simulink model "robot_3axis"  (R2024b)
settings: Solver=ode4  StartTime=0.0  StopTime=simulation_time  FixedStep=Ts  RelTol=1e-3
undefined symbols (not defined in the file): b_r, b_theta, b_z, d_r, d_theta, d_z, dff_r, dff_theta, dff_z, disturbance_time, F_r_max, F_z_max, F_z_min, ff_enable, g, gravity_comp, J_theta, Kd_r, Kd_theta, Kd_z, Ki_r, Ki_theta, Ki_z, Kp_r, Kp_theta, Kp_z, m_r, m_z, move_time, N_filter, noise_r, noise_theta, noise_z, plant_mass_scale, r_final, r_initial, T_theta_max, theta_final, theta_initial, Ts, z_final, z_initial
libraries: slpidlib x3
settings Model: Creator=dell  LastModifiedBy=dell

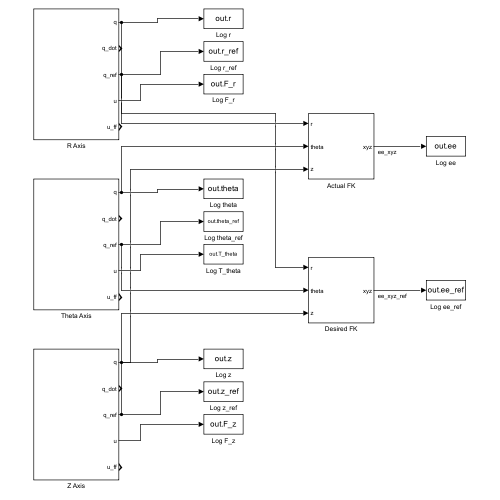
[thumbnail: Simulink's stored preview of the top-level diagram]
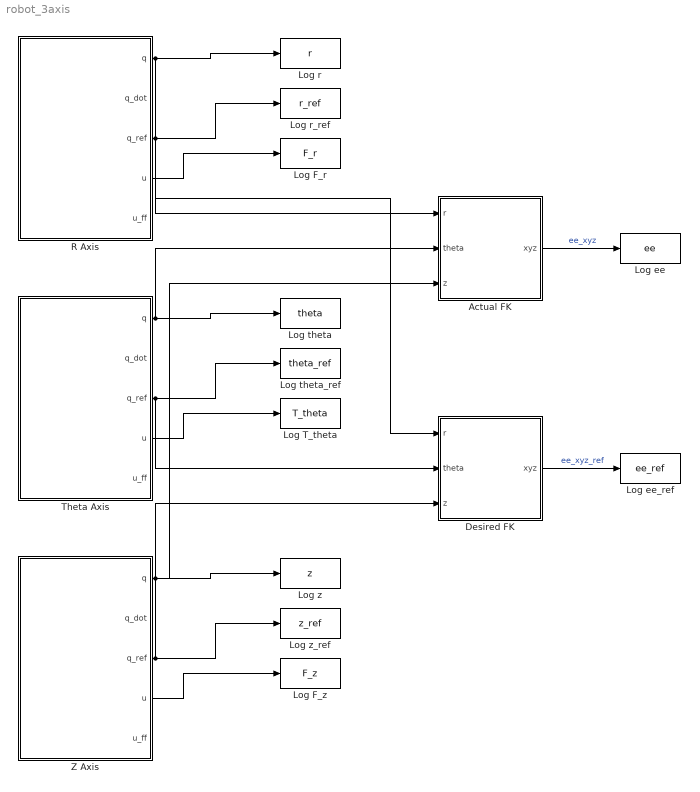
== system robot_3axis ==
  Actual FK : Subsystem
  Desired FK : Subsystem
  Log F_r : ToWorkspace  VariableName=F_r  SaveFormat=Timeseries  SampleTime=-1
  Log F_z : ToWorkspace  VariableName=F_z  SaveFormat=Timeseries  SampleTime=-1
  Log T_theta : ToWorkspace  VariableName=T_theta  SaveFormat=Timeseries  SampleTime=-1
  Log ee : ToWorkspace  VariableName=ee  SaveFormat=Timeseries  SampleTime=-1
  Log ee_ref : ToWorkspace  VariableName=ee_ref  SaveFormat=Timeseries  SampleTime=-1
  Log r : ToWorkspace  VariableName=r  SaveFormat=Timeseries  SampleTime=-1
  Log r_ref : ToWorkspace  VariableName=r_ref  SaveFormat=Timeseries  SampleTime=-1
  Log theta : ToWorkspace  VariableName=theta  SaveFormat=Timeseries  SampleTime=-1
  Log theta_ref : ToWorkspace  VariableName=theta_ref  SaveFormat=Timeseries  SampleTime=-1
  Log z : ToWorkspace  VariableName=z  SaveFormat=Timeseries  SampleTime=-1
  Log z_ref : ToWorkspace  VariableName=z_ref  SaveFormat=Timeseries  SampleTime=-1
  R Axis : Subsystem
  Theta Axis : Subsystem
  Z Axis : Subsystem
  wires:
  R Axis/1(q) -> Log r/1, Actual FK/1(r)
  R Axis/3(q_ref) -> Log r_ref/1, Desired FK/1(r)
  R Axis/4(u) -> Log F_r/1
  Theta Axis/1(q) -> Log theta/1, Actual FK/2(theta)
  Theta Axis/3(q_ref) -> Log theta_ref/1, Desired FK/2(theta)
  Theta Axis/4(u) -> Log T_theta/1
  Z Axis/1(q) -> Log z/1, Actual FK/3(z)
  Z Axis/3(q_ref) -> Log z_ref/1, Desired FK/3(z)
  Z Axis/4(u) -> Log F_z/1
  Actual FK/1(xyz) -> Log ee/1  "ee_xyz"
  Desired FK/1(xyz) -> Log ee_ref/1  "ee_xyz_ref"

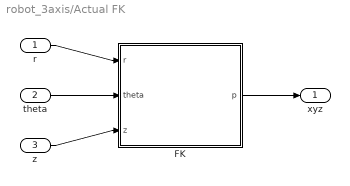
== system robot_3axis/Actual FK ==
  r : Inport
  theta : Inport  Port=2
  z : Inport  Port=3
  FK : MATLAB Function  TreatAsAtomicUnit=on
  xyz : Outport
  wires:
  r/1 -> FK/1(r)
  theta/1 -> FK/2(theta)
  z/1 -> FK/3(z)
  FK/1(p) -> xyz/1

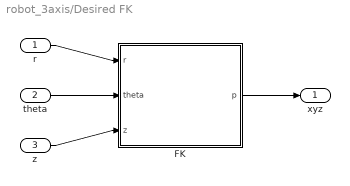
== system robot_3axis/Desired FK ==
  r : Inport
  theta : Inport  Port=2
  z : Inport  Port=3
  FK : MATLAB Function  TreatAsAtomicUnit=on
  xyz : Outport
  wires:
  r/1 -> FK/1(r)
  theta/1 -> FK/2(theta)
  z/1 -> FK/3(z)
  FK/1(p) -> xyz/1

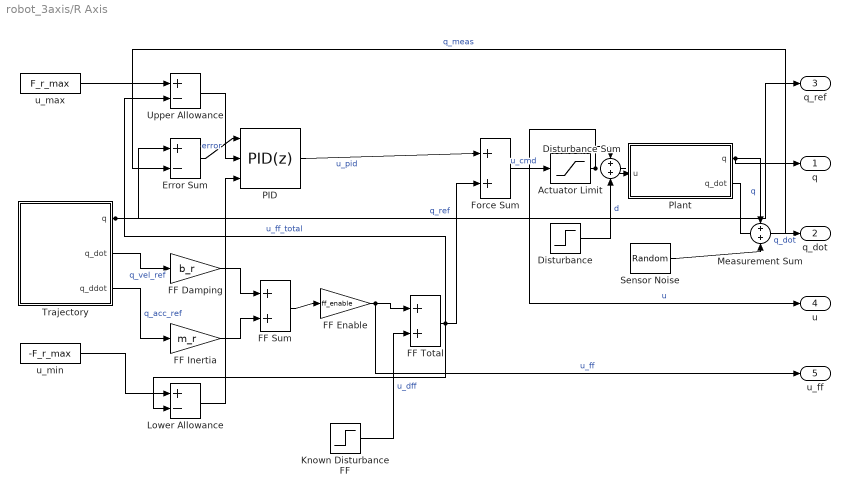
== system robot_3axis/R Axis ==
  Actuator Limit : Saturate  UpperLimit=F_r_max  LowerLimit=-F_r_max
  Disturbance : Step  Time=disturbance_time  After=d_r  SampleTime=0
  Disturbance Sum : Sum
  Error Sum : Sum  Inputs=+-
  FF Damping : Gain  Gain=b_r
  FF Enable : Gain  Gain=ff_enable
  FF Inertia : Gain  Gain=m_r
  FF Sum : Sum
  FF Total : Sum
  Force Sum : Sum
  Known Disturbance FF : Step  Time=disturbance_time  After=dff_r  SampleTime=0
  Lower Allowance : Sum  Inputs=+-
  Measurement Sum : Sum
  PID : slpidlib/PID Controller  Controller=PID  Form=Parallel  TimeDomain=Discrete-time  UseExternalTs=off  SampleTime=Ts  IntegratorMethod=Backward Euler  FilterMethod=Backward Euler  ControllerParametersSource=internal  P=Kp_r  I=Ki_r  UseKiTs=off  D=Kd_r  UseExternalDerivativeSource=off  N=N_filter  UseFilter=off  TunerSelectOption=Transfer Function Based (PID Tuner App)  InitialConditionSource=internal  InitialConditionForIntegrator=0  InitialConditionForFilter=0  DifferentiatorICPrevScaledInput=0  ExternalReset=none  TrackingMode=off  Kt=1  LimitOutput=on  SatLimitsSource=external  UpperSaturationLimit=inf  LowerSaturationLimit=-inf  LinearizeAsGain=off  AntiWindupMode=clamping  Kb=1  LimitIntegrator=off  UpperIntegratorSaturationLimit=inf  LowerIntegratorSaturationLimit=-inf  POutMin=[]  POutMax=[]  IOutMin=[]  IOutMax=[]  DOutMin=[]  DOutMax=[]  NOutMin=[]  NOutMax=[]  SumOutMin=[]  SumOutMax=[]  SaturationOutMin=[]  SaturationOutMax=[]  PParamMin=[]  PParamMax=[]  IParamMin=[]  IParamMax=[]  DParamMin=[]  DParamMax=[]  NParamMin=[]  NParamMax=[]  KbParamMin=[]  KbParamMax=[]  KtParamMin=[]  KtParamMax=[]  KbOutMin=[]  KbOutMax=[]  KtOutMin=[]  KtOutMax=[]  IntegratorOutMin=[]  IntegratorOutMax=[]  FilterOutMin=[]  FilterOutMax=[]  SumI1OutMin=[]  SumI1OutMax=[]  SumI2OutMin=[]  SumI2OutMax=[]  SumI3OutMin=[]  SumI3OutMax=[]  SumI4OutMin=[]  SumI4OutMax=[]  SumDOutMin=[]  SumDOutMax=[]  DifferentiatorOutMin=[]  DifferentiatorOutMax=[]  FilterDiffOutCoefMin=[]  FilterDiffOutCoefMax=[]  ReciprocalOutMin=[]  ReciprocalOutMax=[]  SumDenOutMin=[]  SumDenOutMax=[]  SumNumOutMin=[]  SumNumOutMax=[]  DivideOutMin=[]  DivideOutMax=[]  UdiffTsProdOutMin=[]  UdiffTsProdOutMax=[]  NTsProdOutMin=[]  NTsProdOutMax=[]  UintegralTsProdOutMin=[]  UintegralTsProdOutMax=[]  UngainTsProdOutMin=[]  UngainTsProdOutMax=[]  ClampingZeroOutDataTypeStr=Inherit: Inherit via back propagation  ClampingZeroOutMin=[]  ClampingZeroOutMax=[]  FilterDenConstantOutDataTypeStr=Inherit: Inherit via back propagation  FilterDenConstantOutMin=[]  FilterDenConstantOutMax=[]  PCopyOutDataTypeStr=Inherit: Inherit via back propagation  PCopyOutMin=[]  PCopyOutMax=[]  NCopyOutDataTypeStr=Inherit: Inherit via back propagation  NCopyOutMin=[]  NCopyOutMax=[]  IntegratorContinuousStateAttributes=''  IntegratorStateMustResolveToSignalObject=off  IntegratorRTWStateStorageClass=Auto  FilterContinuousStateAttributes=''  FilterStateMustResolveToSignalObject=off  FilterRTWStateStorageClass=Auto  ParallelPVariant=InternalParameters  IdealPVariant=Disabled  IVariant=InternalParameters  DVariant=InternalParameters  IntegratorVariant=Discrete  SatVariant=External  AWVariant=DiscClampingParallel  PCopyVariant=Disabled  TRVariant=Disabled  FdbkBlocksVariant=Feedback  IdealPFdbkVariant=Passthrough  SatFdbkVariant=Passthrough  DerivativeFilterVariant=Differentiator  NVariant=Passthrough  NCopyVariant=Disabled_SignalSpec  FilterICVariant=InternalICsDifferentiator  IntegratorICVariant=InternalICs  ExternalResetVariant=Disabled  TRSumVariant=Passthrough  SumFdbkVariant=Enabled  SumVariant=Sum_PID  TsampFilterVariant=InternalTs  TsampNgainVariant=Passthrough  TsampIntegralVariant=Disabled_SignalSpec  ExternalSaturationOutDataTypeStr=Inherit: Same as second input  DerivativeSourceVariant=ErrorSignal  PreIntVariant=InternalPreInt
      settings: LibrarySourceBlock=simulink/Discrete/Discrete PID Controller
  Plant : Subsystem
  Sensor Noise : RandomNumber  Variance=noise_r^2  Seed=11  SampleTime=Ts
  Trajectory : Subsystem  mask(Quintic Trajectory){q0=r_initial, qf=r_final, T=move_time}
      mask prompts: q0 "Start position q0"; qf "Final position qf"; T "Duration T (s)"
      mask help: Rest-to-rest quintic trajectory from q0 to qf over T seconds. Outputs position, velocity and acceleration.
      mask Display: disp('Quintic Trajectory')
  Upper Allowance : Sum  Inputs=+-
  u_max : Constant  Value=F_r_max
  u_min : Constant  Value=-F_r_max
  q : Outport
  q_dot : Outport  Port=2
  q_ref : Outport  Port=3
  u : Outport  Port=4
  u_ff : Outport  Port=5
  wires:
  Trajectory/1(q) -> Error Sum/1, q_ref/1  "q_ref"
  Trajectory/2(q_dot) -> FF Damping/1  "q_vel_ref"
  Trajectory/3(q_ddot) -> FF Inertia/1  "q_acc_ref"
  FF Damping/1 -> FF Sum/1
  FF Inertia/1 -> FF Sum/2
  FF Sum/1 -> FF Enable/1
  FF Enable/1 -> FF Total/1, u_ff/1  "u_ff"
  Known Disturbance FF/1 -> FF Total/2  "u_dff"
  Error Sum/1 -> PID/1  "error"
  PID/1 -> Force Sum/1  "u_pid"
  FF Total/1 -> Force Sum/2, Upper Allowance/2, Lower Allowance/2  "u_ff_total"
  u_max/1 -> Upper Allowance/1
  u_min/1 -> Lower Allowance/1
  Upper Allowance/1 -> PID/2
  Lower Allowance/1 -> PID/3
  Force Sum/1 -> Actuator Limit/1  "u_cmd"
  Actuator Limit/1 -> Disturbance Sum/1, u/1  "u"
  Disturbance/1 -> Disturbance Sum/2  "d"
  Disturbance Sum/1 -> Plant/1(u)
  Plant/1(q) -> q/1, Measurement Sum/1  "q"
  Sensor Noise/1 -> Measurement Sum/2
  Measurement Sum/1 -> Error Sum/2  "q_meas"
  Plant/2(q_dot) -> q_dot/1  "q_dot"

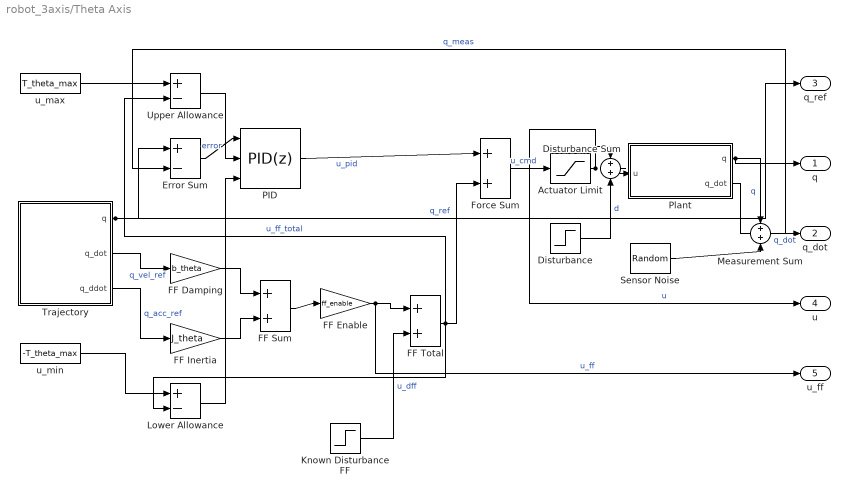
== system robot_3axis/Theta Axis ==
  Actuator Limit : Saturate  UpperLimit=T_theta_max  LowerLimit=-T_theta_max
  Disturbance : Step  Time=disturbance_time  After=d_theta  SampleTime=0
  Disturbance Sum : Sum
  Error Sum : Sum  Inputs=+-
  FF Damping : Gain  Gain=b_theta
  FF Enable : Gain  Gain=ff_enable
  FF Inertia : Gain  Gain=J_theta
  FF Sum : Sum
  FF Total : Sum
  Force Sum : Sum
  Known Disturbance FF : Step  Time=disturbance_time  After=dff_theta  SampleTime=0
  Lower Allowance : Sum  Inputs=+-
  Measurement Sum : Sum
  PID : slpidlib/PID Controller  Controller=PID  Form=Parallel  TimeDomain=Discrete-time  UseExternalTs=off  SampleTime=Ts  IntegratorMethod=Backward Euler  FilterMethod=Backward Euler  ControllerParametersSource=internal  P=Kp_theta  I=Ki_theta  UseKiTs=off  D=Kd_theta  UseExternalDerivativeSource=off  N=N_filter  UseFilter=off  TunerSelectOption=Transfer Function Based (PID Tuner App)  InitialConditionSource=internal  InitialConditionForIntegrator=0  InitialConditionForFilter=0  DifferentiatorICPrevScaledInput=0  ExternalReset=none  TrackingMode=off  Kt=1  LimitOutput=on  SatLimitsSource=external  UpperSaturationLimit=inf  LowerSaturationLimit=-inf  LinearizeAsGain=off  AntiWindupMode=clamping  Kb=1  LimitIntegrator=off  UpperIntegratorSaturationLimit=inf  LowerIntegratorSaturationLimit=-inf  POutMin=[]  POutMax=[]  IOutMin=[]  IOutMax=[]  DOutMin=[]  DOutMax=[]  NOutMin=[]  NOutMax=[]  SumOutMin=[]  SumOutMax=[]  SaturationOutMin=[]  SaturationOutMax=[]  PParamMin=[]  PParamMax=[]  IParamMin=[]  IParamMax=[]  DParamMin=[]  DParamMax=[]  NParamMin=[]  NParamMax=[]  KbParamMin=[]  KbParamMax=[]  KtParamMin=[]  KtParamMax=[]  KbOutMin=[]  KbOutMax=[]  KtOutMin=[]  KtOutMax=[]  IntegratorOutMin=[]  IntegratorOutMax=[]  FilterOutMin=[]  FilterOutMax=[]  SumI1OutMin=[]  SumI1OutMax=[]  SumI2OutMin=[]  SumI2OutMax=[]  SumI3OutMin=[]  SumI3OutMax=[]  SumI4OutMin=[]  SumI4OutMax=[]  SumDOutMin=[]  SumDOutMax=[]  DifferentiatorOutMin=[]  DifferentiatorOutMax=[]  FilterDiffOutCoefMin=[]  FilterDiffOutCoefMax=[]  ReciprocalOutMin=[]  ReciprocalOutMax=[]  SumDenOutMin=[]  SumDenOutMax=[]  SumNumOutMin=[]  SumNumOutMax=[]  DivideOutMin=[]  DivideOutMax=[]  UdiffTsProdOutMin=[]  UdiffTsProdOutMax=[]  NTsProdOutMin=[]  NTsProdOutMax=[]  UintegralTsProdOutMin=[]  UintegralTsProdOutMax=[]  UngainTsProdOutMin=[]  UngainTsProdOutMax=[]  ClampingZeroOutDataTypeStr=Inherit: Inherit via back propagation  ClampingZeroOutMin=[]  ClampingZeroOutMax=[]  FilterDenConstantOutDataTypeStr=Inherit: Inherit via back propagation  FilterDenConstantOutMin=[]  FilterDenConstantOutMax=[]  PCopyOutDataTypeStr=Inherit: Inherit via back propagation  PCopyOutMin=[]  PCopyOutMax=[]  NCopyOutDataTypeStr=Inherit: Inherit via back propagation  NCopyOutMin=[]  NCopyOutMax=[]  IntegratorContinuousStateAttributes=''  IntegratorStateMustResolveToSignalObject=off  IntegratorRTWStateStorageClass=Auto  FilterContinuousStateAttributes=''  FilterStateMustResolveToSignalObject=off  FilterRTWStateStorageClass=Auto  ParallelPVariant=InternalParameters  IdealPVariant=Disabled  IVariant=InternalParameters  DVariant=InternalParameters  IntegratorVariant=Discrete  SatVariant=External  AWVariant=DiscClampingParallel  PCopyVariant=Disabled  TRVariant=Disabled  FdbkBlocksVariant=Feedback  IdealPFdbkVariant=Passthrough  SatFdbkVariant=Passthrough  DerivativeFilterVariant=Differentiator  NVariant=Passthrough  NCopyVariant=Disabled_SignalSpec  FilterICVariant=InternalICsDifferentiator  IntegratorICVariant=InternalICs  ExternalResetVariant=Disabled  TRSumVariant=Passthrough  SumFdbkVariant=Enabled  SumVariant=Sum_PID  TsampFilterVariant=InternalTs  TsampNgainVariant=Passthrough  TsampIntegralVariant=Disabled_SignalSpec  ExternalSaturationOutDataTypeStr=Inherit: Same as second input  DerivativeSourceVariant=ErrorSignal  PreIntVariant=InternalPreInt
      settings: LibrarySourceBlock=simulink/Discrete/Discrete PID Controller
  Plant : Subsystem
  Sensor Noise : RandomNumber  Variance=noise_theta^2  Seed=22  SampleTime=Ts
  Trajectory : Subsystem  mask(Quintic Trajectory){q0=theta_initial, qf=theta_final, T=move_time}
      mask prompts: q0 "Start position q0"; qf "Final position qf"; T "Duration T (s)"
      mask help: Rest-to-rest quintic trajectory from q0 to qf over T seconds. Outputs position, velocity and acceleration.
      mask Display: disp('Quintic Trajectory')
  Upper Allowance : Sum  Inputs=+-
  u_max : Constant  Value=T_theta_max
  u_min : Constant  Value=-T_theta_max
  q : Outport
  q_dot : Outport  Port=2
  q_ref : Outport  Port=3
  u : Outport  Port=4
  u_ff : Outport  Port=5
  wires:
  Trajectory/1(q) -> Error Sum/1, q_ref/1  "q_ref"
  Trajectory/2(q_dot) -> FF Damping/1  "q_vel_ref"
  Trajectory/3(q_ddot) -> FF Inertia/1  "q_acc_ref"
  FF Damping/1 -> FF Sum/1
  FF Inertia/1 -> FF Sum/2
  FF Sum/1 -> FF Enable/1
  FF Enable/1 -> FF Total/1, u_ff/1  "u_ff"
  Known Disturbance FF/1 -> FF Total/2  "u_dff"
  Error Sum/1 -> PID/1  "error"
  PID/1 -> Force Sum/1  "u_pid"
  FF Total/1 -> Force Sum/2, Upper Allowance/2, Lower Allowance/2  "u_ff_total"
  u_max/1 -> Upper Allowance/1
  u_min/1 -> Lower Allowance/1
  Upper Allowance/1 -> PID/2
  Lower Allowance/1 -> PID/3
  Force Sum/1 -> Actuator Limit/1  "u_cmd"
  Actuator Limit/1 -> Disturbance Sum/1, u/1  "u"
  Disturbance/1 -> Disturbance Sum/2  "d"
  Disturbance Sum/1 -> Plant/1(u)
  Plant/1(q) -> q/1, Measurement Sum/1  "q"
  Sensor Noise/1 -> Measurement Sum/2
  Measurement Sum/1 -> Error Sum/2  "q_meas"
  Plant/2(q_dot) -> q_dot/1  "q_dot"

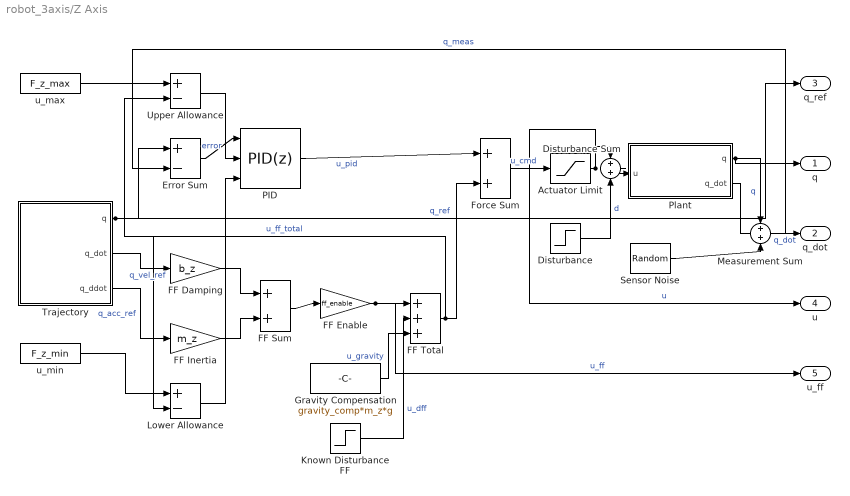
== system robot_3axis/Z Axis ==
  Actuator Limit : Saturate  UpperLimit=F_z_max  LowerLimit=F_z_min
  Disturbance : Step  Time=disturbance_time  After=d_z  SampleTime=0
  Disturbance Sum : Sum
  Error Sum : Sum  Inputs=+-
  FF Damping : Gain  Gain=b_z
  FF Enable : Gain  Gain=ff_enable
  FF Inertia : Gain  Gain=m_z
  FF Sum : Sum
  FF Total : Sum  Inputs=+++
  Force Sum : Sum
  Gravity Compensation : Constant  Value=gravity_comp*m_z*g
  Known Disturbance FF : Step  Time=disturbance_time  After=dff_z  SampleTime=0
  Lower Allowance : Sum  Inputs=+-
  Measurement Sum : Sum
  PID : slpidlib/PID Controller  Controller=PID  Form=Parallel  TimeDomain=Discrete-time  UseExternalTs=off  SampleTime=Ts  IntegratorMethod=Backward Euler  FilterMethod=Backward Euler  ControllerParametersSource=internal  P=Kp_z  I=Ki_z  UseKiTs=off  D=Kd_z  UseExternalDerivativeSource=off  N=N_filter  UseFilter=off  TunerSelectOption=Transfer Function Based (PID Tuner App)  InitialConditionSource=internal  InitialConditionForIntegrator=0  InitialConditionForFilter=0  DifferentiatorICPrevScaledInput=0  ExternalReset=none  TrackingMode=off  Kt=1  LimitOutput=on  SatLimitsSource=external  UpperSaturationLimit=inf  LowerSaturationLimit=-inf  LinearizeAsGain=off  AntiWindupMode=clamping  Kb=1  LimitIntegrator=off  UpperIntegratorSaturationLimit=inf  LowerIntegratorSaturationLimit=-inf  POutMin=[]  POutMax=[]  IOutMin=[]  IOutMax=[]  DOutMin=[]  DOutMax=[]  NOutMin=[]  NOutMax=[]  SumOutMin=[]  SumOutMax=[]  SaturationOutMin=[]  SaturationOutMax=[]  PParamMin=[]  PParamMax=[]  IParamMin=[]  IParamMax=[]  DParamMin=[]  DParamMax=[]  NParamMin=[]  NParamMax=[]  KbParamMin=[]  KbParamMax=[]  KtParamMin=[]  KtParamMax=[]  KbOutMin=[]  KbOutMax=[]  KtOutMin=[]  KtOutMax=[]  IntegratorOutMin=[]  IntegratorOutMax=[]  FilterOutMin=[]  FilterOutMax=[]  SumI1OutMin=[]  SumI1OutMax=[]  SumI2OutMin=[]  SumI2OutMax=[]  SumI3OutMin=[]  SumI3OutMax=[]  SumI4OutMin=[]  SumI4OutMax=[]  SumDOutMin=[]  SumDOutMax=[]  DifferentiatorOutMin=[]  DifferentiatorOutMax=[]  FilterDiffOutCoefMin=[]  FilterDiffOutCoefMax=[]  ReciprocalOutMin=[]  ReciprocalOutMax=[]  SumDenOutMin=[]  SumDenOutMax=[]  SumNumOutMin=[]  SumNumOutMax=[]  DivideOutMin=[]  DivideOutMax=[]  UdiffTsProdOutMin=[]  UdiffTsProdOutMax=[]  NTsProdOutMin=[]  NTsProdOutMax=[]  UintegralTsProdOutMin=[]  UintegralTsProdOutMax=[]  UngainTsProdOutMin=[]  UngainTsProdOutMax=[]  ClampingZeroOutDataTypeStr=Inherit: Inherit via back propagation  ClampingZeroOutMin=[]  ClampingZeroOutMax=[]  FilterDenConstantOutDataTypeStr=Inherit: Inherit via back propagation  FilterDenConstantOutMin=[]  FilterDenConstantOutMax=[]  PCopyOutDataTypeStr=Inherit: Inherit via back propagation  PCopyOutMin=[]  PCopyOutMax=[]  NCopyOutDataTypeStr=Inherit: Inherit via back propagation  NCopyOutMin=[]  NCopyOutMax=[]  IntegratorContinuousStateAttributes=''  IntegratorStateMustResolveToSignalObject=off  IntegratorRTWStateStorageClass=Auto  FilterContinuousStateAttributes=''  FilterStateMustResolveToSignalObject=off  FilterRTWStateStorageClass=Auto  ParallelPVariant=InternalParameters  IdealPVariant=Disabled  IVariant=InternalParameters  DVariant=InternalParameters  IntegratorVariant=Discrete  SatVariant=External  AWVariant=DiscClampingParallel  PCopyVariant=Disabled  TRVariant=Disabled  FdbkBlocksVariant=Feedback  IdealPFdbkVariant=Passthrough  SatFdbkVariant=Passthrough  DerivativeFilterVariant=Differentiator  NVariant=Passthrough  NCopyVariant=Disabled_SignalSpec  FilterICVariant=InternalICsDifferentiator  IntegratorICVariant=InternalICs  ExternalResetVariant=Disabled  TRSumVariant=Passthrough  SumFdbkVariant=Enabled  SumVariant=Sum_PID  TsampFilterVariant=InternalTs  TsampNgainVariant=Passthrough  TsampIntegralVariant=Disabled_SignalSpec  ExternalSaturationOutDataTypeStr=Inherit: Same as second input  DerivativeSourceVariant=ErrorSignal  PreIntVariant=InternalPreInt
      settings: LibrarySourceBlock=simulink/Discrete/Discrete PID Controller
  Plant : Subsystem
  Sensor Noise : RandomNumber  Variance=noise_z^2  Seed=33  SampleTime=Ts
  Trajectory : Subsystem  mask(Quintic Trajectory){q0=z_initial, qf=z_final, T=move_time}
      mask prompts: q0 "Start position q0"; qf "Final position qf"; T "Duration T (s)"
      mask help: Rest-to-rest quintic trajectory from q0 to qf over T seconds. Outputs position, velocity and acceleration.
      mask Display: disp('Quintic Trajectory')
  Upper Allowance : Sum  Inputs=+-
  u_max : Constant  Value=F_z_max
  u_min : Constant  Value=F_z_min
  q : Outport
  q_dot : Outport  Port=2
  q_ref : Outport  Port=3
  u : Outport  Port=4
  u_ff : Outport  Port=5
  wires:
  Trajectory/1(q) -> Error Sum/1, q_ref/1  "q_ref"
  Trajectory/2(q_dot) -> FF Damping/1  "q_vel_ref"
  Trajectory/3(q_ddot) -> FF Inertia/1  "q_acc_ref"
  FF Damping/1 -> FF Sum/1
  FF Inertia/1 -> FF Sum/2
  FF Sum/1 -> FF Enable/1
  FF Enable/1 -> FF Total/1, u_ff/1  "u_ff"
  Known Disturbance FF/1 -> FF Total/2  "u_dff"
  Gravity Compensation/1 -> FF Total/3  "u_gravity"
  Error Sum/1 -> PID/1  "error"
  PID/1 -> Force Sum/1  "u_pid"
  FF Total/1 -> Force Sum/2, Upper Allowance/2, Lower Allowance/2  "u_ff_total"
  u_max/1 -> Upper Allowance/1
  u_min/1 -> Lower Allowance/1
  Upper Allowance/1 -> PID/2
  Lower Allowance/1 -> PID/3
  Force Sum/1 -> Actuator Limit/1  "u_cmd"
  Actuator Limit/1 -> Disturbance Sum/1, u/1  "u"
  Disturbance/1 -> Disturbance Sum/2  "d"
  Disturbance Sum/1 -> Plant/1(u)
  Plant/1(q) -> q/1, Measurement Sum/1  "q"
  Sensor Noise/1 -> Measurement Sum/2
  Measurement Sum/1 -> Error Sum/2  "q_meas"
  Plant/2(q_dot) -> q_dot/1  "q_dot"

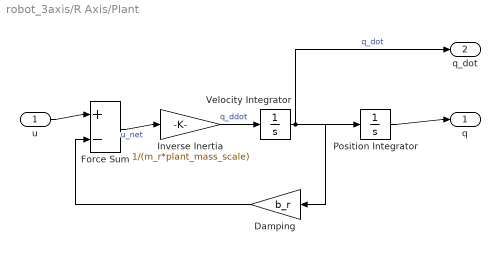
== system robot_3axis/R Axis/Plant ==
  u : Inport
  Damping : Gain  Gain=b_r
  Force Sum : Sum  Inputs=+-
  Inverse Inertia : Gain  Gain=1/(m_r*plant_mass_scale)
  Position Integrator : Integrator  InitialCondition=r_initial
  Velocity Integrator : Integrator
  q : Outport
  q_dot : Outport  Port=2
  wires:
  u/1 -> Force Sum/1
  Force Sum/1 -> Inverse Inertia/1  "u_net"
  Inverse Inertia/1 -> Velocity Integrator/1  "q_ddot"
  Velocity Integrator/1 -> Position Integrator/1, Damping/1, q_dot/1  "q_dot"
  Damping/1 -> Force Sum/2
  Position Integrator/1 -> q/1

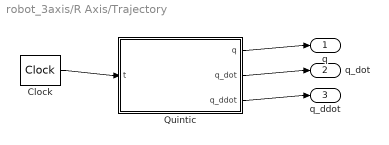
== system robot_3axis/R Axis/Trajectory ==
  Clock : DigitalClock  SampleTime=Ts
  Quintic : MATLAB Function  TreatAsAtomicUnit=on
  q : Outport
  q_dot : Outport  Port=2
  q_ddot : Outport  Port=3
  wires:
  Clock/1 -> Quintic/1(t)
  Quintic/1(q) -> q/1
  Quintic/2(q_dot) -> q_dot/1
  Quintic/3(q_ddot) -> q_ddot/1

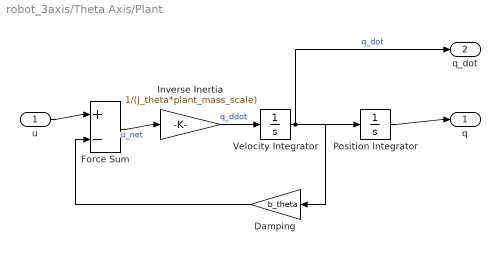
== system robot_3axis/Theta Axis/Plant ==
  u : Inport
  Damping : Gain  Gain=b_theta
  Force Sum : Sum  Inputs=+-
  Inverse Inertia : Gain  Gain=1/(J_theta*plant_mass_scale)
  Position Integrator : Integrator  InitialCondition=theta_initial
  Velocity Integrator : Integrator
  q : Outport
  q_dot : Outport  Port=2
  wires:
  u/1 -> Force Sum/1
  Force Sum/1 -> Inverse Inertia/1  "u_net"
  Inverse Inertia/1 -> Velocity Integrator/1  "q_ddot"
  Velocity Integrator/1 -> Position Integrator/1, Damping/1, q_dot/1  "q_dot"
  Damping/1 -> Force Sum/2
  Position Integrator/1 -> q/1

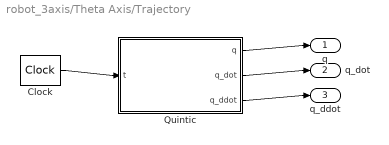
== system robot_3axis/Theta Axis/Trajectory ==
  Clock : DigitalClock  SampleTime=Ts
  Quintic : MATLAB Function  TreatAsAtomicUnit=on
  q : Outport
  q_dot : Outport  Port=2
  q_ddot : Outport  Port=3
  wires:
  Clock/1 -> Quintic/1(t)
  Quintic/1(q) -> q/1
  Quintic/2(q_dot) -> q_dot/1
  Quintic/3(q_ddot) -> q_ddot/1

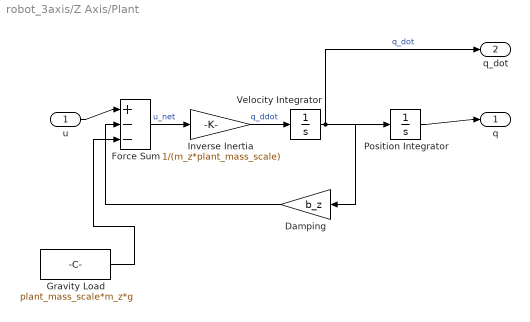
== system robot_3axis/Z Axis/Plant ==
  u : Inport
  Damping : Gain  Gain=b_z
  Force Sum : Sum  Inputs=+--
  Gravity Load : Constant  Value=plant_mass_scale*m_z*g
  Inverse Inertia : Gain  Gain=1/(m_z*plant_mass_scale)
  Position Integrator : Integrator  InitialCondition=z_initial
  Velocity Integrator : Integrator
  q : Outport
  q_dot : Outport  Port=2
  wires:
  u/1 -> Force Sum/1
  Force Sum/1 -> Inverse Inertia/1  "u_net"
  Inverse Inertia/1 -> Velocity Integrator/1  "q_ddot"
  Velocity Integrator/1 -> Position Integrator/1, Damping/1, q_dot/1  "q_dot"
  Damping/1 -> Force Sum/2
  Position Integrator/1 -> q/1
  Gravity Load/1 -> Force Sum/3

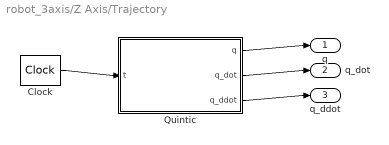
== system robot_3axis/Z Axis/Trajectory ==
  Clock : DigitalClock  SampleTime=Ts
  Quintic : MATLAB Function  TreatAsAtomicUnit=on
  q : Outport
  q_dot : Outport  Port=2
  q_ddot : Outport  Port=3
  wires:
  Clock/1 -> Quintic/1(t)
  Quintic/1(q) -> q/1
  Quintic/2(q_dot) -> q_dot/1
  Quintic/3(q_ddot) -> q_ddot/1

== matlab function robot_3axis/Theta Axis/Trajectory/Quintic ==
  data: t input; q output; q_dot output; q_ddot output; q0 parameter; qf parameter; T parameter
function [q, q_dot, q_ddot] = quintic(t, q0, qf, T)
% Rest-to-rest quintic: zero velocity and acceleration at both ends
tau = min(max(t / T, 0), 1);
d = qf - q0;
q = q0 + d * (10*tau^3 - 15*tau^4 + 6*tau^5);
q_dot = d / T * (30*tau^2 - 60*tau^3 + 30*tau^4);
q_ddot = d / T^2 * (60*tau - 180*tau^2 + 120*tau^3);

== matlab function robot_3axis/R Axis/Trajectory/Quintic ==
  data: t input; q output; q_dot output; q_ddot output; q0 parameter; qf parameter; T parameter
function [q, q_dot, q_ddot] = quintic(t, q0, qf, T)
% Rest-to-rest quintic: zero velocity and acceleration at both ends
tau = min(max(t / T, 0), 1);
d = qf - q0;
q = q0 + d * (10*tau^3 - 15*tau^4 + 6*tau^5);
q_dot = d / T * (30*tau^2 - 60*tau^3 + 30*tau^4);
q_ddot = d / T^2 * (60*tau - 180*tau^2 + 120*tau^3);

== matlab function robot_3axis/Z Axis/Trajectory/Quintic ==
  data: t input; q output; q_dot output; q_ddot output; q0 parameter; qf parameter; T parameter
function [q, q_dot, q_ddot] = quintic(t, q0, qf, T)
% Rest-to-rest quintic: zero velocity and acceleration at both ends
tau = min(max(t / T, 0), 1);
d = qf - q0;
q = q0 + d * (10*tau^3 - 15*tau^4 + 6*tau^5);
q_dot = d / T * (30*tau^2 - 60*tau^3 + 30*tau^4);
q_ddot = d / T^2 * (60*tau - 180*tau^2 + 120*tau^3);

== matlab function robot_3axis/Actual FK/FK ==
  data: r input; p output; theta input; z input
function p = fk(r, theta, z)
% Cylindrical (R-Theta-Z) to Cartesian end-effector position
p = [r * cos(theta); r * sin(theta); z];

== matlab function robot_3axis/Desired FK/FK ==
  data: r input; p output; theta input; z input
function p = fk(r, theta, z)
% Cylindrical (R-Theta-Z) to Cartesian end-effector position
p = [r * cos(theta); r * sin(theta); z];
